simulink model "GainSchedulingSimulinkLookUpTable"  (R2023b)
settings: Solver=VariableStepAuto  StartTime=0.0  StopTime=50.0  RelTol=1e-6
undefined symbols (not defined in the file): K1_sigma, K2_sigma, r, sigma_values
settings Model: Creator=beniaminosquitieri  LastModifiedBy=beniaminosquitieri

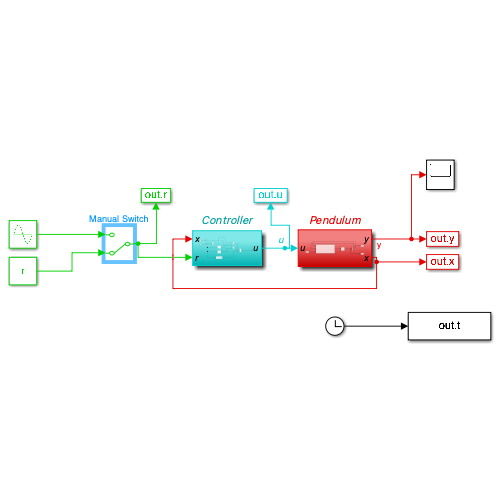
[thumbnail: Simulink's stored preview of the top-level diagram]
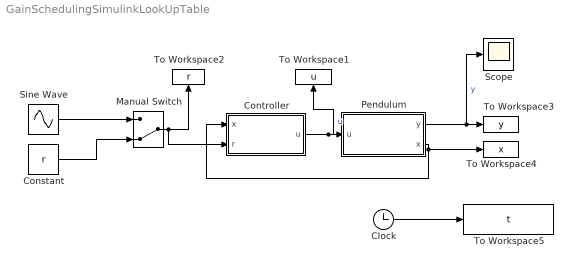
== system GainSchedulingSimulinkLookUpTable ==
  Clock : Clock
  Constant : Constant  Value=r
  Controller : Subsystem
  Manual Switch : ManualSwitch  CurrentSetting=0
  Pendulum : Subsystem
  Scope : Scope
  Sine Wave : Sin  Amplitude=0.5  Frequency=0.1  SampleTime=0
  To Workspace1 : ToWorkspace  VariableName=u  SaveFormat=Timeseries  SampleTime=-1
  To Workspace2 : ToWorkspace  VariableName=r  SaveFormat=Timeseries  SampleTime=-1
  To Workspace3 : ToWorkspace  VariableName=y  SaveFormat=Timeseries  SampleTime=-1
  To Workspace4 : ToWorkspace  VariableName=x  SaveFormat=Timeseries  SampleTime=-1
  To Workspace5 : ToWorkspace  VariableName=t  SaveFormat=Timeseries  SampleTime=-1
  wires:
  Manual Switch/1 -> Controller/2(r), To Workspace2/1
  Pendulum/1(y) -> Scope/1, To Workspace3/1  "y"
  Controller/1(u) -> To Workspace1/1, Pendulum/1(u)  "u"
  Pendulum/2(x) -> Controller/1(x), To Workspace4/1
  Sine Wave/1 -> Manual Switch/1
  Constant/1 -> Manual Switch/2
  Clock/1 -> To Workspace5/1

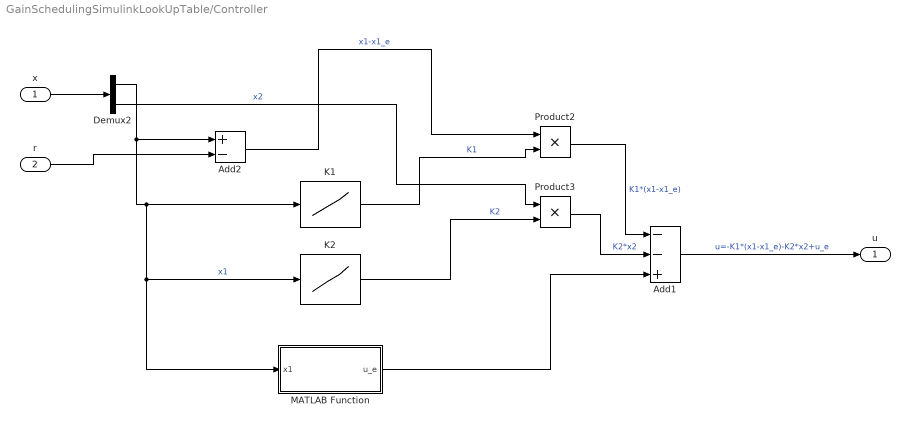
== system GainSchedulingSimulinkLookUpTable/Controller ==
  x : Inport
  r : Inport  Port=2
  Add1 : Sum  Inputs=--+
  Add2 : Sum  Inputs=+-
  Demux2 : Demux  Outputs=2
  K1 : Lookup_n-D  NumberOfTableDimensions=1  BreakpointsForDimension1=sigma_values  Table=K1_sigma  InterpMethod=Cubic spline  InternalRulePriority=Speed  RndMeth=Simplest
  K2 : Lookup_n-D  NumberOfTableDimensions=1  BreakpointsForDimension1=sigma_values  Table=K2_sigma  InterpMethod=Cubic spline  InternalRulePriority=Speed  RndMeth=Simplest
  MATLAB Function : MATLAB Function  TreatAsAtomicUnit=on
  Product2 : Product
  Product3 : Product
  u : Outport
  wires:
  MATLAB Function/1(u_e) -> Add1/3
  x/1 -> Demux2/1
  Product2/1 -> Add1/1  "K1*(x1-x1_e)"
  Demux2/1 -> K1/1, K2/1, MATLAB Function/1(x1), Add2/1  "x1"
  Add1/1 -> u/1  "u=-K1*(x1-x1_e)-K2*x2+u_e"
  Add2/1 -> Product2/1  "x1-x1_e"
  K2/1 -> Product3/2  "K2"
  Demux2/2 -> Product3/1  "x2"
  r/1 -> Add2/2
  K1/1 -> Product2/2  "K1"
  Product3/1 -> Add1/2  "K2*x2"

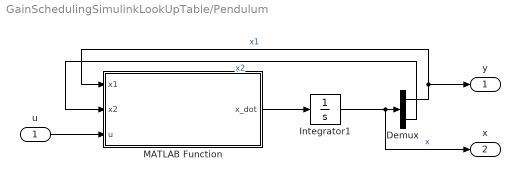
== system GainSchedulingSimulinkLookUpTable/Pendulum ==
  u : Inport
  Demux : Demux  Outputs=2
  Integrator1 : Integrator  InitialCondition=0.0
  MATLAB Function : MATLAB Function  TreatAsAtomicUnit=on
  y : Outport
  x : Outport  Port=2
  wires:
  MATLAB Function/1(x_dot) -> Integrator1/1
  u/1 -> MATLAB Function/3(u)
  Integrator1/1 -> x/1, Demux/1  "x"
  Demux/1 -> MATLAB Function/1(x1), y/1  "x1"
  Demux/2 -> MATLAB Function/2(x2)  "x2"

== matlab function GainSchedulingSimulinkLookUpTable/Controller/MATLAB Function ==
  data: x1 input; u_e output
function u_e = compute_ue(x1)

  
    u_e=-9.81*sin(x1);
   
    
end

== matlab function GainSchedulingSimulinkLookUpTable/Pendulum/MATLAB Function ==
  data: x1 input; x_dot output; x2 input; u input
function x_dot= pendulum_plant(x1, x2, u)

    m = 1; 
    l = 1;
    b = 0.1;
    g = 9.81;
    
    x1_dot = x2;
    x2_dot = (g/l)*sin(x1) - (b/(m*l^2)*x2) + (u/(m*l^2));
    x_dot=[x1_dot,x2_dot];
       
end
